simulink model "h2p3_sim"  (R2021b)
settings: Solver=VariableStepAuto  StartTime=0.0  StopTime=Tf  RelTol=1e-3
undefined symbols (not defined in the file): Cd, H, J, mu, panel, q_inertial2body_0, r0, r_inertial_0, rho0, v_inertial_0, w_b_0
settings Model: Creator=corey  LastModifiedBy=corey

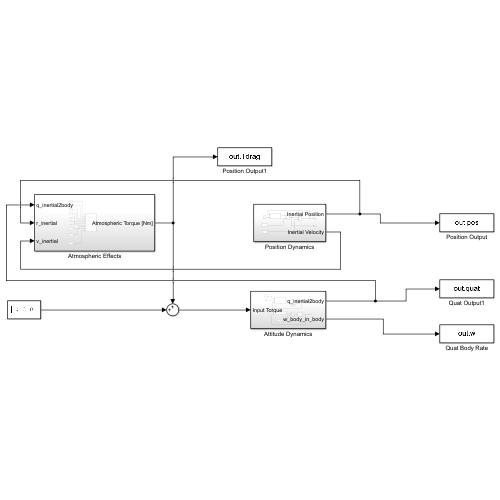
[thumbnail: Simulink's stored preview of the top-level diagram]
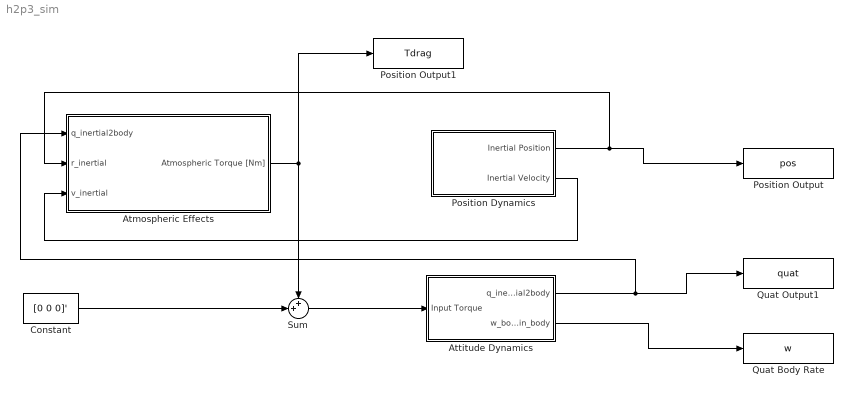
== system h2p3_sim ==
  Atmospheric Effects : Subsystem
  Attitude Dynamics : Subsystem
  Constant : Constant  Value=[0 0 0]'
  Position Dynamics : Subsystem
  Position Output : ToWorkspace  VariableName=pos  SampleTime=-1
  Position Output1 : ToWorkspace  VariableName=Tdrag  SampleTime=-1
  Quat Body Rate : ToWorkspace  VariableName=w  SampleTime=-1
  Quat Output1 : ToWorkspace  VariableName=quat  SampleTime=-1
  Sum : Sum  Inputs=++|
  wires:
  Position Dynamics/1(Inertial Position) -> Atmospheric Effects/2(r_inertial), Position Output/1
  Attitude Dynamics/1(q_inertial2body) -> Atmospheric Effects/1(q_inertial2body), Quat Output1/1
  Attitude Dynamics/2(w_body_in_body) -> Quat Body Rate/1
  Constant/1 -> Sum/2
  Sum/1 -> Attitude Dynamics/1(Input Torque)
  Atmospheric Effects/1(Atmospheric Torque [Nm]) -> Sum/1, Position Output1/1
  Position Dynamics/2(Inertial Velocity) -> Atmospheric Effects/3(v_inertial)

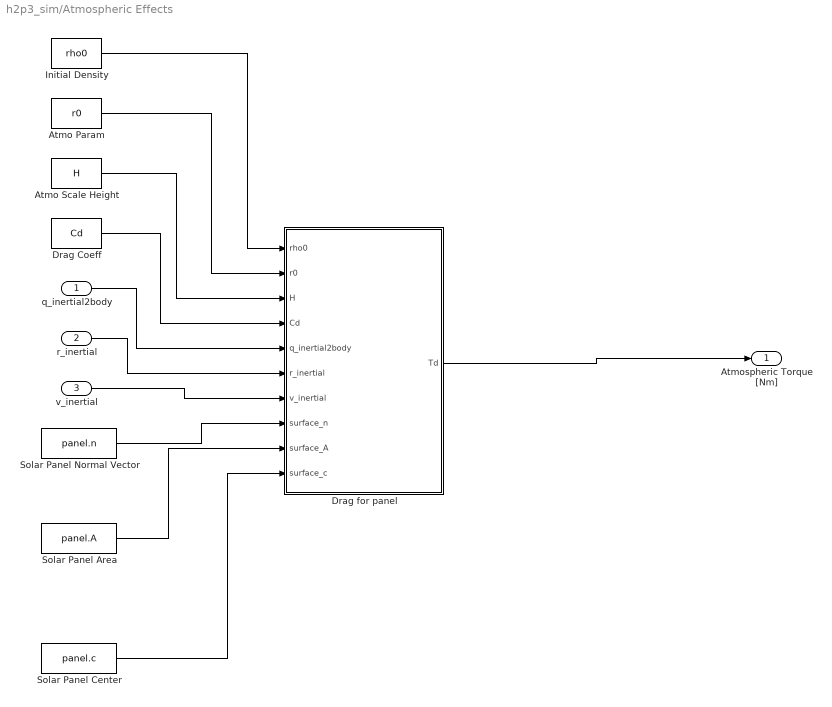
== system h2p3_sim/Atmospheric Effects ==
  q_inertial2body : Inport
  r_inertial : Inport  Port=2
  v_inertial : Inport  Port=3
  Atmo Param : Constant  Value=r0
  Atmo Scale Height : Constant  Value=H
  Drag Coeff : Constant  Value=Cd
  Drag for panel : MATLAB Function  TreatAsAtomicUnit=on
  Initial Density : Constant  Value=rho0
  Solar Panel Area : Constant  Value=panel.A
  Solar Panel Center : Constant  Value=panel.c
  Solar Panel Normal Vector : Constant  Value=panel.n
  Atmospheric Torque [Nm] : Outport
  wires:
  Initial Density/1 -> Drag for panel/1(rho0)
  q_inertial2body/1 -> Drag for panel/5(q_inertial2body)
  r_inertial/1 -> Drag for panel/6(r_inertial)
  v_inertial/1 -> Drag for panel/7(v_inertial)
  Solar Panel Normal Vector/1 -> Drag for panel/8(surface_n)
  Solar Panel Area/1 -> Drag for panel/9(surface_A)
  Drag for panel/1(Td) -> Atmospheric Torque [Nm]/1
  Solar Panel Center/1 -> Drag for panel/10(surface_c)
  Atmo Scale Height/1 -> Drag for panel/3(H)
  Atmo Param/1 -> Drag for panel/2(r0)
  Drag Coeff/1 -> Drag for panel/4(Cd)

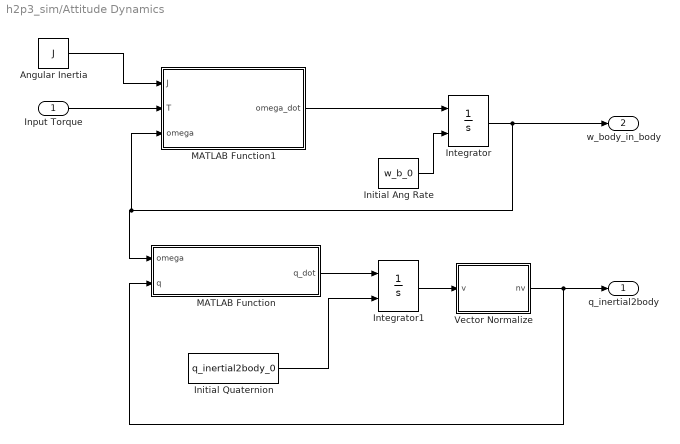
== system h2p3_sim/Attitude Dynamics ==
  Input Torque : Inport
  Angular Inertia : Constant  Value=J
  Initial Ang Rate : Constant  Value=w_b_0
  Initial Quaternion : Constant  Value=q_inertial2body_0
  Integrator : Integrator  InitialConditionSource=external
  Integrator1 : Integrator  InitialConditionSource=external
  MATLAB Function : MATLAB Function  TreatAsAtomicUnit=on
  MATLAB Function1 : MATLAB Function  TreatAsAtomicUnit=on
  Vector Normalize : MATLAB Function  TreatAsAtomicUnit=on
  q_inertial2body : Outport
  w_body_in_body : Outport  Port=2
  wires:
  Integrator/1 -> MATLAB Function1/3(omega), MATLAB Function/1(omega), w_body_in_body/1
  MATLAB Function1/1(omega_dot) -> Integrator/1
  Initial Ang Rate/1 -> Integrator/2
  MATLAB Function/1(q_dot) -> Integrator1/1
  Initial Quaternion/1 -> Integrator1/2
  Integrator1/1 -> Vector Normalize/1(v)
  Vector Normalize/1(nv) -> MATLAB Function/2(q), q_inertial2body/1
  Input Torque/1 -> MATLAB Function1/2(T)
  Angular Inertia/1 -> MATLAB Function1/1(J)

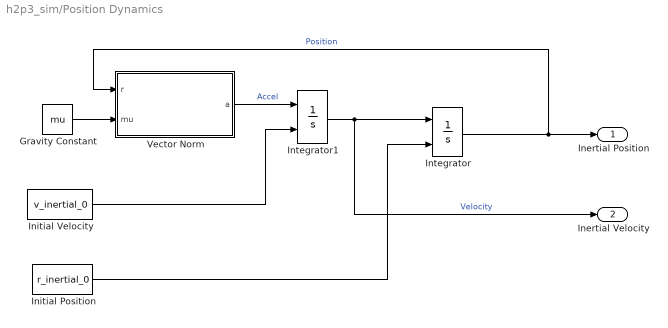
== system h2p3_sim/Position Dynamics ==
  Gravity Constant : Constant  Value=mu
  Initial Position : Constant  Value=r_inertial_0
  Initial Velocity : Constant  Value=v_inertial_0
  Integrator : Integrator  InitialConditionSource=external  InitialCondition=[6871, 0, 0]'
  Integrator1 : Integrator  InitialConditionSource=external  InitialCondition=[0, 7.6166, 0]'
  Vector Norm : MATLAB Function  TreatAsAtomicUnit=on
  Inertial Position : Outport
  Inertial Velocity : Outport  Port=2
  wires:
  Integrator/1 -> Vector Norm/1(r), Inertial Position/1  "Position"
  Integrator1/1 -> Inertial Velocity/1, Integrator/1  "Velocity"
  Vector Norm/1(a) -> Integrator1/1  "Accel"
  Gravity Constant/1 -> Vector Norm/2(mu)
  Initial Velocity/1 -> Integrator1/2
  Initial Position/1 -> Integrator/2

== matlab function h2p3_sim/Attitude Dynamics/MATLAB Function ==
  data: omega input; q_dot output; q input
function q_dot = QuaternionEvolution(omega, q)
intermed = [omega; 0];
q_dot = 0.5*QuatProduct(intermed,q);

== matlab function h2p3_sim/Position Dynamics/Vector Norm ==
  data: r input; a output; mu input
function a = TwoBodyGrav(r,mu)

nr = norm(r);
a = -mu*r/(nr^3);

== matlab function h2p3_sim/Attitude Dynamics/MATLAB Function1 ==
  data: J input; omega_dot output; T input; omega input
function omega_dot = OmegaEvolution(J, T, omega)
omega_dot = J\(T - cross(omega, J*omega));

== matlab function h2p3_sim/Attitude Dynamics/Vector Normalize ==
  data: v input; nv output
function nv = NormVec(v)

nv = v/norm(v);

== matlab function h2p3_sim/Atmospheric Effects/Drag for panel ==
  data: Td output; rho0 input; r0 input; H input; Cd input; q_inertial2body input; r_inertial input; v_inertial input; surface_n input; surface_A input; surface_c input
function Td = DragTorque(rho0, r0, H, Cd, q_inertial2body, r_inertial, v_inertial, surface_n, surface_A, surface_c)

% Find the velocity of the atmosphere
w_earth = 7.3E-5; % rad/sec
v_atmo = [-w_earth*r_inertial(2), w_earth*r_inertial(1), 0]';
v_rel = 1000*(v_inertial - v_atmo); % 1000 factor to convert to m/s
v_rel_hat = v_rel/norm(v_rel);

% Atmospheric density with exponential model
rhoA = rho0*exp(-(norm(r_inertial) - r0)/H);

% Rotate surface normal into inertial frame
surface_n_inertial = QuatTransform(QuatInv(q_inertial2body),surface_n);

% Force in inertial frame
Fd = -0.5*Cd*rhoA*norm(v_rel)^2*(surface_n_inertial'*v_rel_hat)*v_rel_hat*surface_A;

% Rotate
Fd_body = QuatTransform(q_inertial2body,Fd);

% Torque in the body
Td = cross(Fd_body, surface_c);
